simulink model "TST_FlCDspl_DD"  (R2016b)
settings: Solver=FixedStepDiscrete  StartTime=0.0  StopTime=simTime  FixedStep=sampleTime  RelTol=1e-3
values from neighbouring files (symbols this model uses):
  testCase = 1    [initTST_FlCDspl_DD_001.m]
libraries: simulink x2
settings Model: Creator=Wei Liang  LastModifiedBy=Wei Liang
settings DebuggingCC: SignalRangeChecking=error

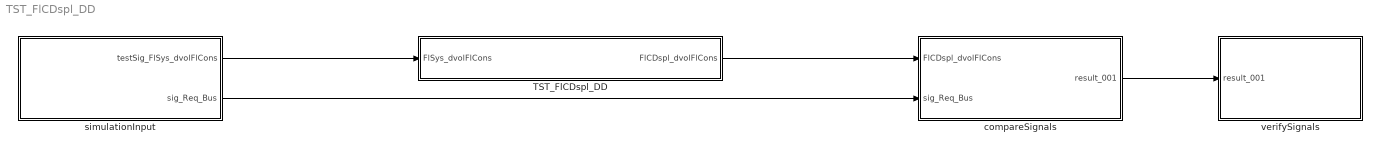
== system TST_FlCDspl_DD ==
  TST_FlCDspl_DD : Subsystem
  compareSignals : Subsystem
  simulationInput : Subsystem
  verifySignals : Subsystem
  wires:
  simulationInput/1(testSig_FlSys_dvolFlCons) -> TST_FlCDspl_DD/1(FlSys_dvolFlCons)
  TST_FlCDspl_DD/1(FlCDspl_dvolFlCons) -> compareSignals/1(FlCDspl_dvolFlCons)
  simulationInput/2(sig_Req_Bus) -> compareSignals/2(sig_Req_Bus)
  compareSignals/1(result_001) -> verifySignals/1(result_001)

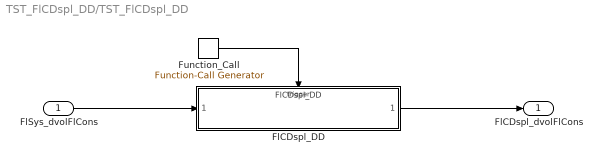
== system TST_FlCDspl_DD/TST_FlCDspl_DD ==
  FlSys_dvolFlCons : Inport
  FlCDspl_DD : ModelReference  ModelNameDialog=FlCDspl_DD  ModelReferenceVersion=1.18  TriggerPortName=function  TriggerPortTriggerType=function-call  TriggerPortStatesWhenEnabling=held
  Function_Call : simulink/Ports & Subsystems/Function-Call Generator  sample_time=sampleTime  numberOfIterations=1
  FlCDspl_dvolFlCons : Outport
  wires:
  Function_Call/1 -> FlCDspl_DD/Trigger
  FlSys_dvolFlCons/1 -> FlCDspl_DD/1
  FlCDspl_DD/1 -> FlCDspl_dvolFlCons/1

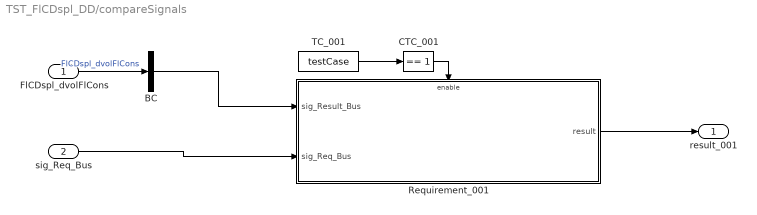
== system TST_FlCDspl_DD/compareSignals ==
  FlCDspl_dvolFlCons : Inport
  sig_Req_Bus : Inport  Port=2
  BC : BusCreator  Inputs=1
  CTC_001 : simulink/Logic and Bit Operations/Compare To Constant  relop===  const=1  OutDataTypeStr=boolean
  Requirement_001 : Subsystem
  TC_001 : Constant  Value=testCase
  result_001 : Outport
  wires:
  FlCDspl_dvolFlCons/1 -> BC/1  "FlCDspl_dvolFlCons"
  TC_001/1 -> CTC_001/1
  CTC_001/1 -> Requirement_001/Enable
  sig_Req_Bus/1 -> Requirement_001/2(sig_Req_Bus)
  BC/1 -> Requirement_001/1(sig_Result_Bus)
  Requirement_001/1(result) -> result_001/1

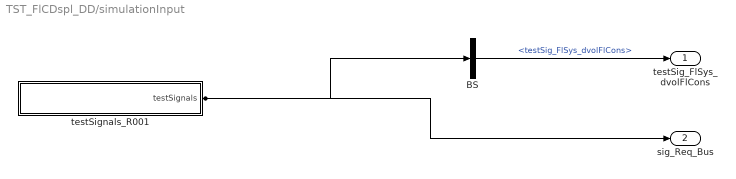
== system TST_FlCDspl_DD/simulationInput ==
  BS : BusSelector  OutputSignals=testSig_FlSys_dvolFlCons
  testSignals_R001 : Subsystem
  testSig_FlSys_dvolFlCons : Outport
  sig_Req_Bus : Outport  Port=2
  wires:
  BS/1 -> testSig_FlSys_dvolFlCons/1  "<testSig_FlSys_dvolFlCons>"
  testSignals_R001/1(testSignals) -> BS/1, sig_Req_Bus/1

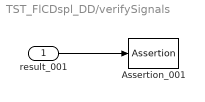
== system TST_FlCDspl_DD/verifySignals ==
  result_001 : Inport
  Assertion_001 : Assertion  Enabled=off
  wires:
  result_001/1 -> Assertion_001/1

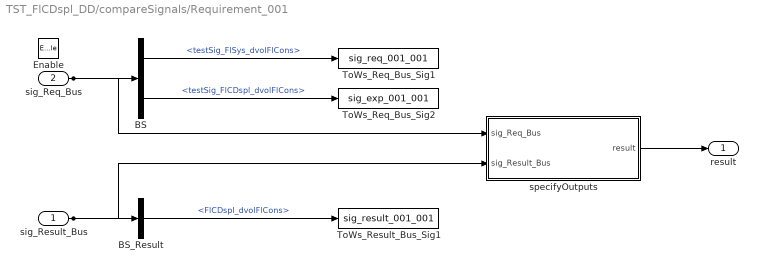
== system TST_FlCDspl_DD/compareSignals/Requirement_001 ==
  sig_Result_Bus : Inport
  sig_Req_Bus : Inport  Port=2
  Enable : EnablePort
  BS : BusSelector  OutputSignals=testSig_FlSys_dvolFlCons,testSig_FlCDspl_dvolFlCons
  BS_Result : BusSelector  OutputSignals=FlCDspl_dvolFlCons
  ToWs_Req_Bus_Sig1 : ToWorkspace  VariableName=sig_req_001_001  SaveFormat=Structure With Time
  ToWs_Req_Bus_Sig2 : ToWorkspace  VariableName=sig_exp_001_001  SaveFormat=Structure With Time
  ToWs_Result_Bus_Sig1 : ToWorkspace  VariableName=sig_result_001_001  SaveFormat=Structure With Time
  specifyOutputs : Subsystem
  result : Outport
  wires:
  sig_Req_Bus/1 -> BS/1, specifyOutputs/1(sig_Req_Bus)
  BS/1 -> ToWs_Req_Bus_Sig1/1  "<testSig_FlSys_dvolFlCons>"
  BS/2 -> ToWs_Req_Bus_Sig2/1  "<testSig_FlCDspl_dvolFlCons>"
  sig_Result_Bus/1 -> BS_Result/1, specifyOutputs/2(sig_Result_Bus)
  BS_Result/1 -> ToWs_Result_Bus_Sig1/1  "<FlCDspl_dvolFlCons>"
  specifyOutputs/1(result) -> result/1

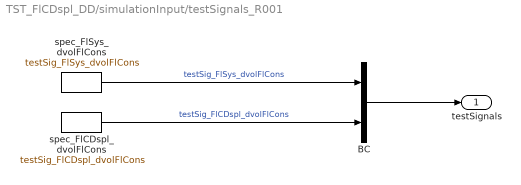
== system TST_FlCDspl_DD/simulationInput/testSignals_R001 ==
  BC : BusCreator  Inputs=2
  spec_FlCDspl_dvolFlCons : FromWorkspace  VariableName=testSig_FlCDspl_dvolFlCons  Interpolate=off  OutputAfterFinalValue=Holding final value
  spec_FlSys_dvolFlCons : FromWorkspace  VariableName=testSig_FlSys_dvolFlCons  Interpolate=off  OutputAfterFinalValue=Holding final value
  testSignals : Outport
  wires:
  BC/1 -> testSignals/1
  spec_FlSys_dvolFlCons/1 -> BC/1  "testSig_FlSys_dvolFlCons"
  spec_FlCDspl_dvolFlCons/1 -> BC/2  "testSig_FlCDspl_dvolFlCons"

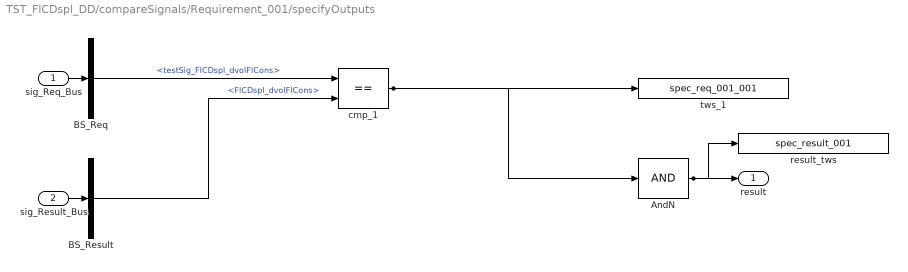
== system TST_FlCDspl_DD/compareSignals/Requirement_001/specifyOutputs ==
  sig_Req_Bus : Inport
  sig_Result_Bus : Inport  Port=2
  AndN : Logic  Inputs=1
  BS_Req : BusSelector  OutputSignals=testSig_FlCDspl_dvolFlCons
  BS_Result : BusSelector  OutputSignals=FlCDspl_dvolFlCons
  cmp_1 : RelationalOperator  Operator===  RndMeth=Nearest  InputSameDT=on
  result_tws : ToWorkspace  VariableName=spec_result_001
  tws_1 : ToWorkspace  VariableName=spec_req_001_001
  result : Outport
  wires:
  sig_Req_Bus/1 -> BS_Req/1
  sig_Result_Bus/1 -> BS_Result/1
  AndN/1 -> result/1, result_tws/1
  BS_Req/1 -> cmp_1/1  "<testSig_FlCDspl_dvolFlCons>"
  BS_Result/1 -> cmp_1/2  "<FlCDspl_dvolFlCons>"
  cmp_1/1 -> tws_1/1, AndN/1
